simulink model "untitled"  (R2020a)
settings: Solver=VariableStepAuto  StartTime=0.0  StopTime=10.0  RelTol=1e-3
settings Model: Creator=Marwan Mohamed  LastModifiedBy=Marwan Mohamed

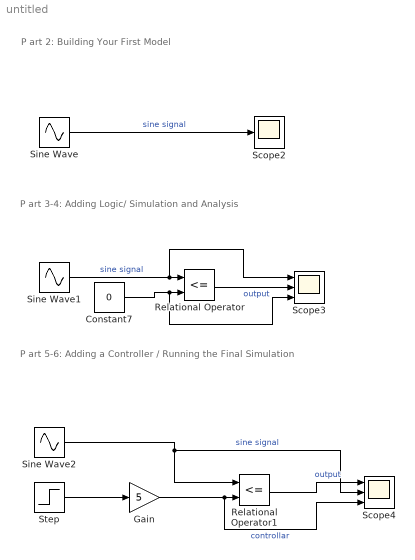
== system untitled ==
  note: P art 5-6: Adding a Controller / Running the Final Simulation
  note: P art 3-4: Adding Logic/ Simulation and Analysis
  note: P art 2: Building Your First Model
  Constant7 : Constant  Value=0
  Gain : Gain  Gain=5
  Relational Operator : RelationalOperator  Operator=<=  OutDataTypeStr=boolean  RndMeth=Simplest
  Relational Operator1 : RelationalOperator  Operator=<=  OutDataTypeStr=boolean  RndMeth=Simplest
  Scope2 : Scope
  Scope3 : Scope  NumInputPorts=3
  Scope4 : Scope  NumInputPorts=3
  Sine Wave : Sin  SampleTime=0
  Sine Wave1 : Sin  SampleTime=0
  Sine Wave2 : Sin  SampleTime=0
  Step : Step  SampleTime=2
  wires:
  Sine Wave/1 -> Scope2/1  "sine signal"
  Sine Wave1/1 -> Scope3/1, Relational Operator/1  "sine signal"
  Constant7/1 -> Scope3/3, Relational Operator/2
  Relational Operator/1 -> Scope3/2  "output"
  Sine Wave2/1 -> Scope4/2, Relational Operator1/1  "sine signal"
  Step/1 -> Gain/1
  Gain/1 -> Scope4/3, Relational Operator1/2  "controllar"
  Relational Operator1/1 -> Scope4/1  "output"
